simulink model "mech_conveyor"  (Simulink 7.1)
settings: Solver=ode45  StartTime=0  StopTime=inf  FixedStep=0.1  RelTol=1e-4  AbsTol=1e-6
PreLoadFcn:
  | load mech_conveyor_controller;
InitFcn:
  | mech_slider_open(gcs)
values from neighbouring files (symbols this model uses):
  Ak = [-1697.70247289 -84.8146549606 -57.1718135112 270.473316945 -57.171813483 12.9581182618 -530032.227354 -51423.5874655 -37197.2166541 203871.174251 -37141.5821622 18540.2571033 ... (324 elements, 18x18)]    [mech_stewart_control_Hinf.mat]
  Aw = [0 0 0 0 0 0 0 0 0 0 0 0 ... (36 elements, 6x6)]    [mech_stewart_control_Hinf.mat]
  Bk = [1697.70247289 84.8146549606 57.1718135112 -270.473316945 57.171813483 -12.9581182618 444258.815048 42487.6011968 30423.7625952 -164792.340046 30370.0437282 -14348.6043858 ... (216 elements, 18x12)]    [mech_stewart_control_Hinf.mat]
  Bw = [3162.27766017 0 0 0 0 0 0 3162.27766017 0 0 0 0 ... (36 elements, 6x6)]    [mech_stewart_control_Hinf.mat]
  Ck = [-1.00011609263 5.97678206219e-05 3.18868867016e-05 -2.514712894e-05 7.64338569004e-06 -9.44720298065e-06 -9.44724487133e-06 7.6433999019e-06 -2.51471714827e-05 3.18868934787e-05 5.97678371914e-05 -1.00011609263 ... (108 elements, 6x18)]    [mech_stewart_control_Hinf.mat]
  Cw = [3162.27766017 0 0 0 0 0 0 3162.27766017 0 0 0 0 ... (36 elements, 6x6)]    [mech_stewart_control_Hinf.mat]
  Dk = [0 0 0 0 0 0 0 0 0 0 0 0 ... (72 elements, 6x12)]    [mech_stewart_control_Hinf.mat]
  Dw = [40000000 0 0 0 0 0 0 40000000 0 0 0 0 ... (36 elements, 6x6)]    [mech_stewart_control_Hinf.mat]
undefined symbols (not defined in the file or in its folder): Awinv, Bwinv, Cwinv, Dwinv
libraries: mblibv1 x18, simulink x1
settings Model: Creator=arnav  LastModifiedBy=batserve  ExtModeAutoUpdateStatusClock=off
settings DataIOCC: SignalLoggingName=sigsOut
settings OptimizationCC: BooleanDataType=off  InlineInvariantSignals=on
settings DebuggingCC: AlgebraicLoopMsg=none  SaveWithParameterizedLinksMsg=none  CheckExecutionContextPreStartOutputMsg=on  CheckExecutionContextRuntimeOutputMsg=on  SignalResolutionControl=TryResolveAllWithWarning  SolverPrmCheckMsg=none  MultiTaskDSMMsg=warning  MultiTaskCondExecSysMsg=none  UnconnectedInputMsg=none  UnconnectedOutputMsg=none  UnconnectedLineMsg=none  StrictBusMsg=None
settings HardwareCC: TargetBitPerLong=64  TargetEndianess=LittleEndian  TargetWordSize=64  TargetHWDeviceType=MATLAB Host  ProdEqTarget=off
settings RTWCC: SystemTargetFile=rsim.tlc  TemplateMakefile=rsim_default_tmf  Description=Rapid Simulation Target  ProcessScript=rsim_make_rtw_hook  IncludeERTFirstTime=on
settings RSimTargetCC: TargetFcnLib=ansi_tfl_tmw.mat  TargetFunctionLibrary=ANSI_C  IsPILTarget=off  EnableShiftOperators=on  PortableWordSizes=off
settings SimMechanicsCC: WarnOnRedundantConstraints=off

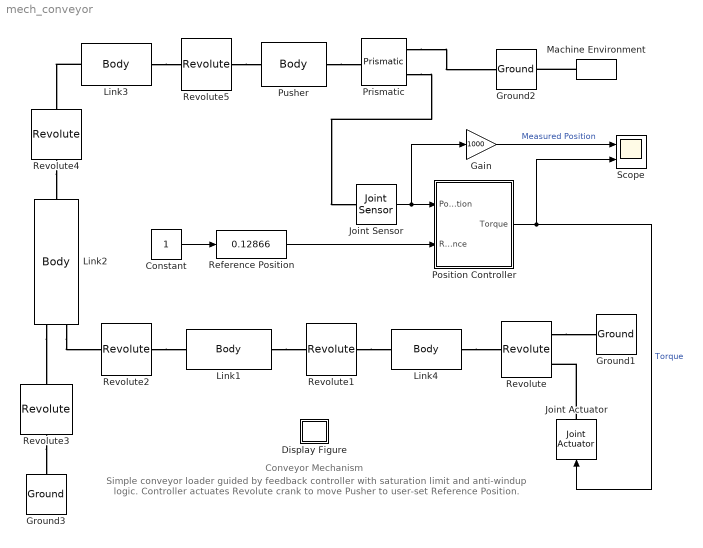
== system mech_conveyor ==
  note: Conveyor Mechanism
  note: Simple conveyor loader guided by feedback controller with saturation limit
      | and anti-windup logic. Controller actuates Revolute crank to move Pusher
      | to user-set Reference Position.
  Constant : Constant  OutDataType=sfix(16)  OutScaling=2^0
  Display Figure : Subsystem  Tag=Help  Description="Help callback for conveyor model: mech_conveyor.  Opens Help browser to Type 19 marker at documentation for this tutorial model."
      settings: OpenFcn=helpview([docroot '/toolbox/physmod/mech/mech.map'], 'mech_conveyor_help');
      mask Type: Help callback
      mask Display: image(imread('info.bmp'))
  Gain : Gain  Gain=1000  ParameterDataType=sfix(16)  ParameterScaling=2^0  OutDataType=sfix(16)  OutScaling=2^0  SaturateOnIntegerOverflow=on  OutDataTypeStr=Inherit: Same as input  ParamDataTypeStr=Inherit: Same as input
  Ground1 : mblibv1/Bodies/Ground  Orientation=left  DialogController=MECH.DynMechDlgSource  SystemSampleTime=-1  LeftPortType=env  RightPortType=workingframe  PhysicalDomain=Mechanical  DialogClass=GroundBlock  CoordPosition=[0.280 0.210 0]  CoordPositionUnits=m  StateVectorMgrId=-1  MachineId=[0 0]  ShowEnvPort=off
  Ground2 : mblibv1/Bodies/Ground  Orientation=left  DialogController=MECH.DynMechDlgSource  SystemSampleTime=-1  LeftPortType=env  RightPortType=workingframe  PhysicalDomain=Mechanical  DialogClass=GroundBlock  CoordPosition=[0.412 0.5 0]  CoordPositionUnits=m  StateVectorMgrId=-1  MachineId=[0 0]  ShowEnvPort=on
  Ground3 : mblibv1/Bodies/Ground  Orientation=up  DialogController=MECH.DynMechDlgSource  SystemSampleTime=-1  LeftPortType=env  RightPortType=workingframe  PhysicalDomain=Mechanical  DialogClass=GroundBlock  CoordPosition=[0.08 0.11 0]  CoordPositionUnits=m  StateVectorMgrId=-1  MachineId=[0 0]  ShowEnvPort=off
  Joint Actuator : mblibv1/Sensors &  Actuators/Joint Actuator  Orientation=up  DialogController=MECH.DynMechDlgSource  SystemSampleTime=-1  PhysicalDomain=Mechanical  PortType=blob  ActuationStyle=Force  AngleUnits=rad  ArcVelocityUnits=rad/s  ArcAccelerationUnits=rad/s^2  CoordPositionUnits=m  VelocityUnits=m/s  AccelerationUnits=m/s^2  ForceUnits=N  TorqueUnits=N-m  ActiveIO=on  Width=1  DialogClass=MechanicalActuatorBlock  Primitive=R1  ReferenceFrame=Absolute (INERTIAL)
  Joint Sensor : mblibv1/Sensors &  Actuators/Joint Sensor  DialogController=MECH.DynMechDlgSource  SystemSampleTime=-1  PhysicalDomain=Mechanical  PortType=blob  Muxed=on  Pose=off  Angle=on  AngleUnits=deg  ArcVelocity=off  ArcVelocityUnits=deg/s  ArcAcceleration=off  ArcAccelerationUnits=deg/s^2  CoordPosition=on  CoordPositionUnits=m  Velocity=off  VelocityUnits=m/s  Acceleration=off  AccelerationUnits=m/s^2  Quaternion=on  QuaternionDT=off  QuaternionDDT=off  QuaternionUnits=off  OutputVector=[ 1 ]  ActiveIO=on  Width=1  DialogClass=MechanicalSensorBlock  Primitive=P1  Force=off  ForceUnits=N  Torque=off  TorqueUnits=N-m  ReferenceFrame=Absolute (INERTIAL)  ReactionSensedSide=Base  ReactionReferenceFrame=Absolute (World)  ReactionForce=off  ReactionForceUnits=N  ReactionMoment=off  ReactionMomentUnits=N-m
  Link1 : mblibv1/Bodies/Body  Orientation=left  DialogController=MECH.DynMechDlgSource  PhysicalDomain=mechanical  SubClassName=Unknown  LeftPortType=workingframe  RightPortType=workingframe  LConnTagsString=CS1  RConnTagsString=CS2  DialogClass=MechanicalBodyBlock  Mass=0.98785  MassUnits=kg  InertiaUnits=kg*m^2  Inertia=[7.6414e-005 -9.2222e-005 1.8971e-009;-9.2222e-005 0.0083286 -2.5235e-010;1.8971e-009 -2.5235e-010 0.0083397]  Shape=Cylinder  ShapeDims=[1 1]  ShapeUnits=m  ShapeUse=false  Density=1  DensityUnits=kg/m^3  DensityUse=false  GraphicsMode=1  BodyColor=[0.5 0.5 0.5]  GraphicsObj=[]  AttachedToCS=1  CG=Left$CG$[0.110 0.247 0]$WORLD$WORLD$m$[0 0 -4.22]$Euler X-Y-Z$deg$WORLD$false  WorkingFrames=Left$CS1$[0.265 0.236 0]$WORLD$WORLD$m$[0 0 0]$Euler X-Y-Z$deg$WORLD$true#Right$CS2$[-0.299 0.022 0]$WORLD$CS1$m$[0 0 0]$Euler X-Y-Z$deg$WORLD$true  CGPos=[0.110 0.247 0]  CGRot=[0 0 -4.22]  CS0Pos=[]  CS0Rot=[]  CS1Pos=[0.265 0.236 0]  CS1Rot=[0 0 0]  CS2Pos=[-0.299 0.022 0]  CS2Rot=[0 0 0]  CS3Pos=[]  CS3Rot=[]  CS4Pos=[]  CS4Rot=[]  CS5Pos=[]  CS5Rot=[]  CS6Pos=[]  CS6Rot=[]  CS7Pos=[]  CS7Rot=[]  CS8Pos=[]  CS8Rot=[]  CS9Pos=[]  CS9Rot=[]  CS10Pos=[]  CS10Rot=[]  CS11Pos=[]  CS11Rot=[]  CS12Pos=[]  CS12Rot=[]  CS13Pos=[]  CS13Rot=[]  CS14Pos=[]  CS14Rot=[]  CS15Pos=[]  CS15Rot=[]  CS16Pos=[]  CS16Rot=[]  CS17Pos=[]  CS17Rot=[]  CS18Pos=[]  CS18Rot=[]  CS19Pos=[]  CS19Rot=[]  CS20Pos=[]  CS20Rot=[]
  Link2 : mblibv1/Bodies/Body  Orientation=up  DialogController=MECH.DynMechDlgSource  PhysicalDomain=mechanical  SubClassName=Unknown  LeftPortType=workingframe  RightPortType=workingframe  LConnTagsString=CS1|CS2  RConnTagsString=CS3  DialogClass=MechanicalBodyBlock  Mass=2.7433  MassUnits=kg  InertiaUnits=kg*m^2  Inertia=[0.0044915 2.9472e-005 1.0996e-007;2.9472e-005 0.089001 -4.3534e-007;1.0996e-007 -4.3534e-007 0.093312]  Shape=Cylinder  ShapeDims=[1 1]  ShapeUnits=m  ShapeUse=false  Density=1  DensityUnits=kg/m^3  DensityUse=false  GraphicsMode=1  BodyColor=[0.5 0.5 0.5]  GraphicsObj=[]  AttachedToCS=1  CG=Left$CG$[-0.030 0.402 0]$WORLD$WORLD$m$[0 0 95.31]$Euler X-Y-Z$deg$WORLD$false  WorkingFrames=Left$CS1$[0.08 0.11 0]$WORLD$WORLD$m$[0 0 0]$Euler X-Y-Z$deg$WORLD$true#Left$CS2$[-0.114 0.148 0]$WORLD$CS1$m$[0 0 0]$Euler X-Y-Z$deg$WORLD$true#Right$CS3$[0.059 0.449 0]$WORLD$CS2$m$[0 0 0]$Euler X-Y-Z$deg$WORLD$true  CGPos=[-0.030 0.402 0]  CGRot=[0 0 95.31]  CS0Pos=[]  CS0Rot=[]  CS1Pos=[0.08 0.11 0]  CS1Rot=[0 0 0]  CS2Pos=[-0.114 0.148 0]  CS2Rot=[0 0 0]  CS3Pos=[0.059 0.449 0]  CS3Rot=[0 0 0]  CS4Pos=[]  CS4Rot=[]  CS5Pos=[]  CS5Rot=[]  CS6Pos=[]  CS6Rot=[]  CS7Pos=[]  CS7Rot=[]  CS8Pos=[]  CS8Rot=[]  CS9Pos=[]  CS9Rot=[]  CS10Pos=[]  CS10Rot=[]  CS11Pos=[]  CS11Rot=[]  CS12Pos=[]  CS12Rot=[]  CS13Pos=[]  CS13Rot=[]  CS14Pos=[]  CS14Rot=[]  CS15Pos=[]  CS15Rot=[]  CS16Pos=[]  CS16Rot=[]  CS17Pos=[]  CS17Rot=[]  CS18Pos=[]  CS18Rot=[]  CS19Pos=[]  CS19Rot=[]  CS20Pos=[]  CS20Rot=[]
  Link3 : mblibv1/Bodies/Body  DialogController=MECH.DynMechDlgSource  PhysicalDomain=mechanical  SubClassName=Unknown  LeftPortType=workingframe  RightPortType=workingframe  LConnTagsString=CS1  RConnTagsString=CS2  DialogClass=MechanicalBodyBlock  Mass=1.2355  MassUnits=kg  InertiaUnits=kg*m^2  Inertia=[8.2129e-005 1.8216e-005 -3.7069e-010;1.8216e-005 0.017391 -2.6914e-011;-3.7069e-010 -2.6914e-011 0.017392]  Shape=Cylinder  ShapeDims=[1 1]  ShapeUnits=m  ShapeUse=false  Density=1  DensityUnits=kg/m^3  DensityUse=false  GraphicsMode=1  BodyColor=[0.5 0.5 0.5]  GraphicsObj=[]  AttachedToCS=1  CG=Left$CG$[0.194 0.604 0.01]$WORLD$WORLD$m$[90 -31.24 0]$Euler X-Y-Z$deg$WORLD$false  WorkingFrames=Left$CS1$[0.025 0.707 0]$WORLD$WORLD$m$[0 0 0]$Euler X-Y-Z$deg$WORLD$true#Right$CS2$[0.342 -0.207 0]$WORLD$CS1$m$[0 0 0]$Euler X-Y-Z$deg$WORLD$true  CGPos=[0.194 0.604 0.01]  CGRot=[90 -31.24 0]  CS0Pos=[]  CS0Rot=[]  CS1Pos=[0.025 0.707 0]  CS1Rot=[0 0 0]  CS2Pos=[0.342 -0.207 0]  CS2Rot=[0 0 0]  CS3Pos=[]  CS3Rot=[]  CS4Pos=[]  CS4Rot=[]  CS5Pos=[]  CS5Rot=[]  CS6Pos=[]  CS6Rot=[]  CS7Pos=[]  CS7Rot=[]  CS8Pos=[]  CS8Rot=[]  CS9Pos=[]  CS9Rot=[]  CS10Pos=[]  CS10Rot=[]  CS11Pos=[]  CS11Rot=[]  CS12Pos=[]  CS12Rot=[]  CS13Pos=[]  CS13Rot=[]  CS14Pos=[]  CS14Rot=[]  CS15Pos=[]  CS15Rot=[]  CS16Pos=[]  CS16Rot=[]  CS17Pos=[]  CS17Rot=[]  CS18Pos=[]  CS18Rot=[]  CS19Pos=[]  CS19Rot=[]  CS20Pos=[]  CS20Rot=[]
  Link4 : mblibv1/Bodies/Body  Orientation=left  DialogController=MECH.DynMechDlgSource  PhysicalDomain=mechanical  SubClassName=Unknown  LeftPortType=workingframe  RightPortType=workingframe  LConnTagsString=CS1  RConnTagsString=CS2  DialogClass=MechanicalBodyBlock  Mass=0.057538  MassUnits=kg  InertiaUnits=kg*m^2  Inertia=[1.0148e-005 0 0;0 2.5218e-006 0;0 0 1.1711e-005]  Shape=Cylinder  ShapeDims=[1 1]  ShapeUnits=m  ShapeUse=false  Density=1  DensityUnits=kg/m^3  DensityUse=false  GraphicsMode=1  BodyColor=[0.5 0.5 0.5]  GraphicsObj=[]  AttachedToCS=1  CG=Left$CG$[0.272 0.223 0.01]$WORLD$WORLD$m$[0 0 30]$Euler X-Y-Z$deg$WORLD$false  WorkingFrames=Left$CS1$[0.280 0.210 0]$WORLD$WORLD$m$[0 0 0]$Euler X-Y-Z$deg$WORLD$true#Right$CS2$[-0.015 0.026 0]$CS1$CS1$m$[0 0 0]$Euler X-Y-Z$deg$WORLD$true  CGPos=[0.272 0.223 0.01]  CGRot=[0 0 30]  CS0Pos=[]  CS0Rot=[]  CS1Pos=[0.280 0.210 0]  CS1Rot=[0 0 0]  CS2Pos=[-0.015 0.026 0]  CS2Rot=[0 0 0]  CS3Pos=[]  CS3Rot=[]  CS4Pos=[]  CS4Rot=[]  CS5Pos=[]  CS5Rot=[]  CS6Pos=[]  CS6Rot=[]  CS7Pos=[]  CS7Rot=[]  CS8Pos=[]  CS8Rot=[]  CS9Pos=[]  CS9Rot=[]  CS10Pos=[]  CS10Rot=[]  CS11Pos=[]  CS11Rot=[]  CS12Pos=[]  CS12Rot=[]  CS13Pos=[]  CS13Rot=[]  CS14Pos=[]  CS14Rot=[]  CS15Pos=[]  CS15Rot=[]  CS16Pos=[]  CS16Rot=[]  CS17Pos=[]  CS17Rot=[]  CS18Pos=[]  CS18Rot=[]  CS19Pos=[]  CS19Rot=[]  CS20Pos=[]  CS20Rot=[]
  Machine Environment : mblibv1/Bodies/Machine Environment  Tag=Factory ground  Orientation=left  DialogController=MECH.DialogSource  SystemSampleTime=-1  PortType=env  PhysicalDomain=Mechanical  DialogTemplateClass=MECH.MachineEnvironment  SyncWhenCopied=off  Gravity=[0 -9.81 0]  GravityUnits=m/s^2  GravityAsSignal=off  Dimensionality=3D Only  AnalysisType=Forward dynamics  LinearAssemblyTolerance=1e-3  LinearAssemblyToleranceUnits=m  AngularAssemblyTolerance=1e-3  AngularAssemblyToleranceUnits=rad  ConstraintSolverType=Stabilizing  ConstraintRelTolerance=1e-4  ConstraintAbsTolerance=1e-4  UseRobustSingularityHandling=off  RedundancyAnalysisToleranceType=Automatically select tolerance  RedundancyAnalysisTolerance=1e-14  StatePerturbationType=Adaptive  PerturbationSize=1e-3  VisualizeMachine=on
  Position Controller : Subsystem
  Prismatic : mblibv1/Joints/Prismatic  Orientation=left  DialogController=MECH.DynMechDlgSource  PhysicalDomain=mechanical  SubClassName=Unknown  LeftPortType=blob  RightPortType=blob  LConnTagsString=__newl0|SA1  RConnTagsString=__newr0  NumSAPorts=1  CutJoint=off  MarkAsCut=off  Primitives=prismatic  PrimitiveProps=P1$WORLD$[1 0 0]$prismatic  DialogClass=JointBlock  P1Axis=[1 0 0]
  Pusher : mblibv1/Bodies/Body  DialogController=MECH.DynMechDlgSource  PhysicalDomain=mechanical  SubClassName=Unknown  LeftPortType=workingframe  RightPortType=workingframe  LConnTagsString=CS1  RConnTagsString=CS2  DialogClass=MechanicalBodyBlock  Mass=1.8547  MassUnits=kg  InertiaUnits=kg*m^2  Inertia=[0.0025031 -1.671e-006 5.5014e-006;-1.671e-006 0.0016406 -1.8596e-007;5.5014e-006 -1.8596e-007 0.0011862]  Shape=Cylinder  ShapeDims=[1 1]  ShapeUnits=m  ShapeUse=false  Density=1  DensityUnits=kg/m^3  DensityUse=false  GraphicsMode=1  BodyColor=[0.5 0.5 0.5]  GraphicsObj=[]  AttachedToCS=1  CG=Left$CG$[0.396 0.499 0]$WORLD$WORLD$m$[0 0 0]$Euler X-Y-Z$deg$WORLD$false  WorkingFrames=Left$CS1$[0.367 0.5 0]$WORLD$WORLD$m$[0 0 0]$Euler X-Y-Z$deg$WORLD$true#Right$CS2$[0.045 0 0]$WORLD$CS1$m$[0 0 0]$Euler X-Y-Z$deg$WORLD$true  CGPos=[0.396 0.499 0]  CGRot=[0 0 0]  CS0Pos=[]  CS0Rot=[]  CS1Pos=[0.367 0.5 0]  CS1Rot=[0 0 0]  CS2Pos=[0.045 0 0]  CS2Rot=[0 0 0]  CS3Pos=[]  CS3Rot=[]  CS4Pos=[]  CS4Rot=[]  CS5Pos=[]  CS5Rot=[]  CS6Pos=[]  CS6Rot=[]  CS7Pos=[]  CS7Rot=[]  CS8Pos=[]  CS8Rot=[]  CS9Pos=[]  CS9Rot=[]  CS10Pos=[]  CS10Rot=[]  CS11Pos=[]  CS11Rot=[]  CS12Pos=[]  CS12Rot=[]  CS13Pos=[]  CS13Rot=[]  CS14Pos=[]  CS14Rot=[]  CS15Pos=[]  CS15Rot=[]  CS16Pos=[]  CS16Rot=[]  CS17Pos=[]  CS17Rot=[]  CS18Pos=[]  CS18Rot=[]  CS19Pos=[]  CS19Rot=[]  CS20Pos=[]  CS20Rot=[]
  Reference Position : simulink/Math Operations/Slider Gain  Tag="685  662  330   98"  SystemSampleTime=-1  low=0  gain=0.12866  high=0.2
  Revolute : mblibv1/Joints/Revolute  Orientation=left  DialogController=MECH.DynMechDlgSource  PhysicalDomain=mechanical  SubClassName=Unknown  LeftPortType=blob  RightPortType=blob  LConnTagsString=__newl0|SA1  RConnTagsString=__newr0  NumSAPorts=1  CutJoint=off  MarkAsCut=off  Primitives=revolute  PrimitiveProps=R1$WORLD$[0 0 1]$revolute  DialogClass=JointBlock  R1Axis=[0 0 1]
  Revolute1 : mblibv1/Joints/Revolute  Orientation=left  DialogController=MECH.DynMechDlgSource  PhysicalDomain=mechanical  SubClassName=Unknown  LeftPortType=blob  RightPortType=blob  LConnTagsString=__newl0  RConnTagsString=__newr0  NumSAPorts=0  CutJoint=off  MarkAsCut=off  Primitives=revolute  PrimitiveProps=R1$WORLD$[0 0 1]$revolute  DialogClass=JointBlock  R1Axis=[0 0 1]
  Revolute2 : mblibv1/Joints/Revolute  Orientation=left  DialogController=MECH.DynMechDlgSource  PhysicalDomain=mechanical  SubClassName=Unknown  LeftPortType=blob  RightPortType=blob  LConnTagsString=__newl0  RConnTagsString=__newr0  NumSAPorts=0  CutJoint=on  MarkAsCut=off  Primitives=revolute  PrimitiveProps=R1$WORLD$[0 0 1]$revolute  DialogClass=JointBlock  R1Axis=[0 0 1]
  Revolute3 : mblibv1/Joints/Revolute  Orientation=up  DialogController=MECH.DynMechDlgSource  PhysicalDomain=mechanical  SubClassName=Unknown  LeftPortType=blob  RightPortType=blob  LConnTagsString=__newl0  RConnTagsString=__newr0  NumSAPorts=0  CutJoint=off  MarkAsCut=off  Primitives=revolute  PrimitiveProps=R1$WORLD$[0 0 1]$revolute  DialogClass=JointBlock  R1Axis=[0 0 1]
  Revolute4 : mblibv1/Joints/Revolute  Orientation=up  DialogController=MECH.DynMechDlgSource  PhysicalDomain=mechanical  SubClassName=Unknown  LeftPortType=blob  RightPortType=blob  LConnTagsString=__newl0  RConnTagsString=__newr0  NumSAPorts=0  CutJoint=on  MarkAsCut=off  Primitives=revolute  PrimitiveProps=R1$WORLD$[0 0 1]$revolute  DialogClass=JointBlock  R1Axis=[0 0 1]
  Revolute5 : mblibv1/Joints/Revolute  DialogController=MECH.DynMechDlgSource  PhysicalDomain=mechanical  SubClassName=Unknown  LeftPortType=blob  RightPortType=blob  LConnTagsString=__newl0  RConnTagsString=__newr0  NumSAPorts=0  CutJoint=off  MarkAsCut=off  Primitives=revolute  PrimitiveProps=R1$WORLD$[0 0 1]$revolute  DialogClass=JointBlock  R1Axis=[0 0 1]
  Scope : Scope  NumInputPorts=2
      settings: TimeRange=20  YMin=-50~-4  YMax=250~4
  wires:
  Joint Sensor/1 -> Position Controller/1(Position), Gain/1
  Constant/1 -> Reference Position/1
  Position Controller/1(Torque) -> Joint Actuator/1, Scope/2  "Torque"
  Reference Position/1 -> Position Controller/2(Reference)
  Gain/1 -> Scope/1  "Measured Position"
  connections:
  Link2/LConn1 -- Revolute3/RConn1
  Revolute3/LConn1 -- Ground3/RConn1
  Revolute4/LConn1 -- Link2/RConn1
  Link2/LConn2 -- Revolute2/RConn1
  Link3/LConn1 -- Revolute4/RConn1
  Link3/RConn1 -- Revolute5/LConn1
  Revolute5/RConn1 -- Pusher/LConn1
  Revolute2/LConn1 -- Link1/RConn1
  Link1/LConn1 -- Revolute1/RConn1
  Revolute1/LConn1 -- Link4/RConn1
  Link4/LConn1 -- Revolute/RConn1
  Revolute/LConn1 -- Ground1/RConn1
  Prismatic/LConn2 -- Joint Sensor/LConn1
  Joint Actuator/RConn1 -- Revolute/LConn2
  Prismatic/LConn1 -- Ground2/RConn1
  Pusher/RConn1 -- Prismatic/RConn1
  Machine Environment/RConn1 -- Ground2/LConn1

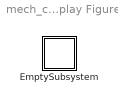
== system mech_conveyor/Display Figure ==
  EmptySubsystem : Subsystem

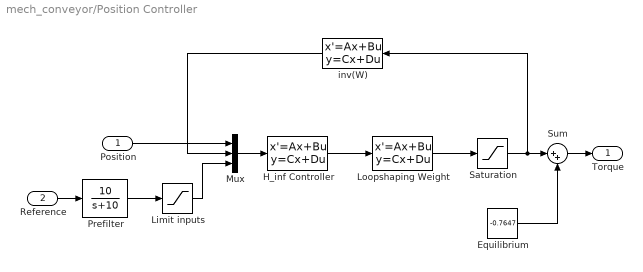
== system mech_conveyor/Position Controller ==
  Position : Inport  OutDataType=sfix(16)  OutScaling=2^0
  Reference : Inport  Port=2  OutDataType=sfix(16)  OutScaling=2^0
  Equilibrium : Constant  Value=-0.7647  OutDataType=sfix(16)  OutScaling=2^0
  H_inf Controller : StateSpace  A=Ak  B=Bk  C=Ck  D=Dk
  Limit inputs : Saturate  UpperLimit=0.2  LowerLimit=0
  Loopshaping Weight : StateSpace  A=Aw  B=Bw  C=Cw  D=Dw
  Mux : Mux  Inputs=3
  Prefilter : TransferFcn  Numerator=[10]  Denominator=[1 10]
  Saturation : Saturate  UpperLimit=5  LowerLimit=-5+0.7647
  Sum : Sum  Inputs=|++  OutDataType=sfix(16)  OutScaling=2^0  SaturateOnIntegerOverflow=on  InputSameDT=on  OutDataTypeStr=Inherit: Same as first input
  inv(W) : StateSpace  Orientation=left  A=Awinv  B=Bwinv  C=Cwinv  D=Dwinv
  Torque : Outport  OutDataType=sfix(16)  OutScaling=2^0
  wires:
  H_inf Controller/1 -> Loopshaping Weight/1
  Mux/1 -> H_inf Controller/1
  Position/1 -> Mux/1
  Limit inputs/1 -> Mux/3
  inv(W)/1 -> Mux/2
  Loopshaping Weight/1 -> Saturation/1
  Saturation/1 -> Sum/1, inv(W)/1
  Sum/1 -> Torque/1
  Equilibrium/1 -> Sum/2
  Prefilter/1 -> Limit inputs/1
  Reference/1 -> Prefilter/1

== system mech_conveyor/Display Figure/EmptySubsystem ==
